simulink model "Q1a_Q1b_Helicopter_System"  (R2020a)
settings: Solver=VariableStepAuto  StartTime=0.0  StopTime=100  MaxStep=0.01  RelTol=1e-3
settings Model: Creator=Ajita Shree  LastModifiedBy=Ajita Shree

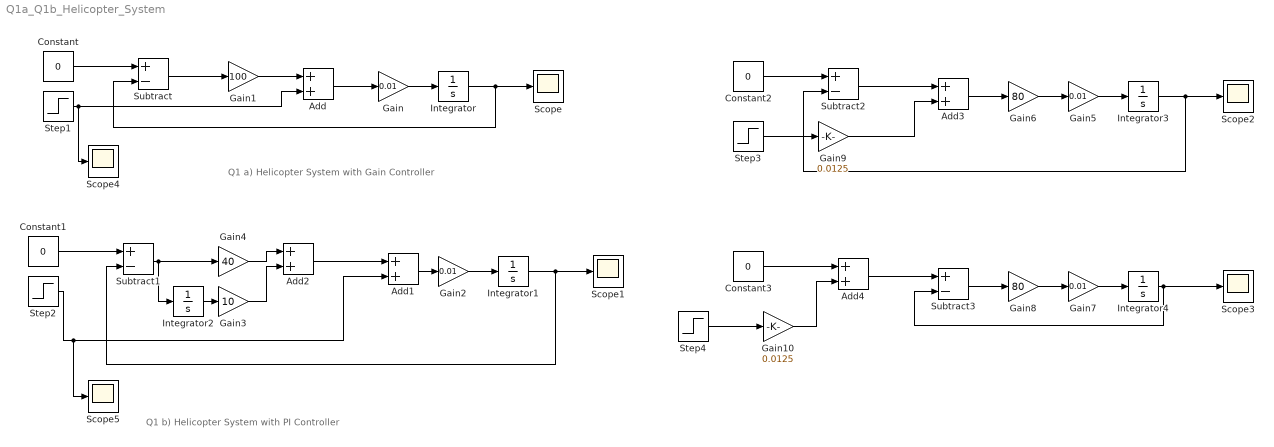
== system Q1a_Q1b_Helicopter_System ==
  note: Q1 b) Helicopter System with PI Controller
  note: Q1 a) Helicopter System with Gain Controller
  Add{,1..4} (5 alike) : Sum
  Constant{,1..3} (4 alike) : Constant  Value=0
  Gain{,2,5,7} (4 alike) : Gain  Gain=0.01
  Gain1 : Gain  Gain=100
  Gain10 : Gain  Gain=0.0125
  Gain3 : Gain  Gain=10
  Gain4 : Gain  Gain=40
  Gain6 : Gain  Gain=80
  Gain8 : Gain  Gain=80
  Gain9 : Gain  Gain=0.0125
  Integrator{,1..4} (5 alike) : Integrator
  Scope{,1..5} (6 alike) : Scope
  Step{1..4} (4 alike) : Step  Time=5  SampleTime=0
  Subtract{,1..3} (4 alike) : Sum  Inputs=+-
  wires:
  Gain/1 -> Integrator/1
  Constant/1 -> Subtract/1
  Integrator/1 -> Subtract/2, Scope/1
  Subtract/1 -> Gain1/1
  Gain1/1 -> Add/1
  Add/1 -> Gain/1
  Step1/1 -> Scope4/1, Add/2
  Subtract1/1 -> Integrator2/1, Gain4/1
  Gain2/1 -> Integrator1/1
  Constant1/1 -> Subtract1/1
  Add2/1 -> Add1/1
  Integrator1/1 -> Subtract1/2, Scope1/1
  Step2/1 -> Scope5/1, Add1/2
  Add1/1 -> Gain2/1
  Gain4/1 -> Add2/1
  Gain3/1 -> Add2/2
  Integrator2/1 -> Gain3/1
  Gain5/1 -> Integrator3/1
  Constant2/1 -> Subtract2/1
  Integrator3/1 -> Subtract2/2, Scope2/1
  Step3/1 -> Gain9/1
  Subtract2/1 -> Add3/1
  Add3/1 -> Gain6/1
  Gain9/1 -> Add3/2
  Gain6/1 -> Gain5/1
  Step4/1 -> Gain10/1
  Gain8/1 -> Gain7/1
  Integrator4/1 -> Subtract3/2, Scope3/1
  Subtract3/1 -> Gain8/1
  Gain7/1 -> Integrator4/1
  Constant3/1 -> Add4/1
  Add4/1 -> Subtract3/1
  Gain10/1 -> Add4/2
